simulink model "Lab5sim"  (R2023a)
settings: Solver=FixedStepAuto  StartTime=0.0  StopTime=tOut(end)  FixedStep=dt  RelTol=1e-3
values from neighbouring files (symbols this model uses):
  den = [(C*R) 1 (R/L)]    [t1_final.m]    (also in t2_final.m)
  num = [1 0]    [t1_final.m]    (also in t2_final.m)
undefined symbols (not defined in the file or in its folder): dt
settings Model: Creator=sucho  LastModifiedBy=sucho

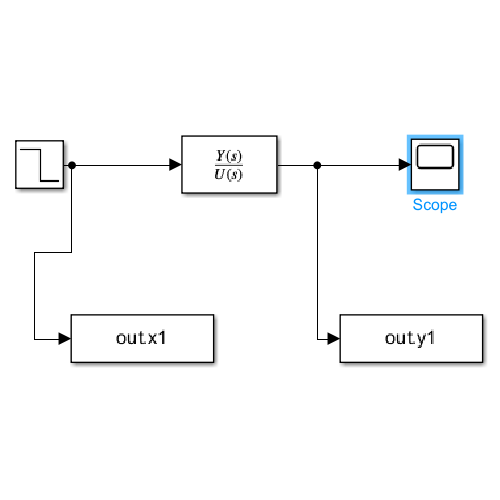
[thumbnail: Simulink's stored preview of the top-level diagram]
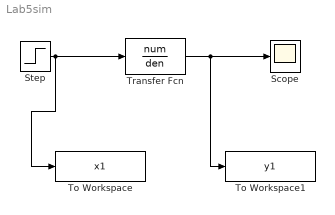
== system Lab5sim ==
  Scope : Scope
  Step : Step  Time=dt  Before=1  After=0  SampleTime=0
  To Workspace : ToWorkspace  VariableName=x1  SaveFormat=Timeseries  SampleTime=-1
  To Workspace1 : ToWorkspace  VariableName=y1  SaveFormat=Timeseries  SampleTime=-1
  Transfer Fcn : TransferFcn  Numerator=num  Denominator=den
  wires:
  Step/1 -> To Workspace/1, Transfer Fcn/1
  Transfer Fcn/1 -> To Workspace1/1, Scope/1
